simulink model "SignalGen"  (R2014a)
settings: Solver=ode45  StartTime=0.0  StopTime=inf  RelTol=1e-3
undefined symbols (not defined in the file or in its folder): f, Tsample
libraries: dspxfrm3 x3, dspsrcs4 x2, dsparch4 x1, dspsigops x1, commnoisgen2 x1
settings Model: Creator=pHysiX  LastModifiedBy=MrBigBear
settings DebuggingCC: UnderspecifiedInitializationDetection=Classic  StateNameClashWarn=warning

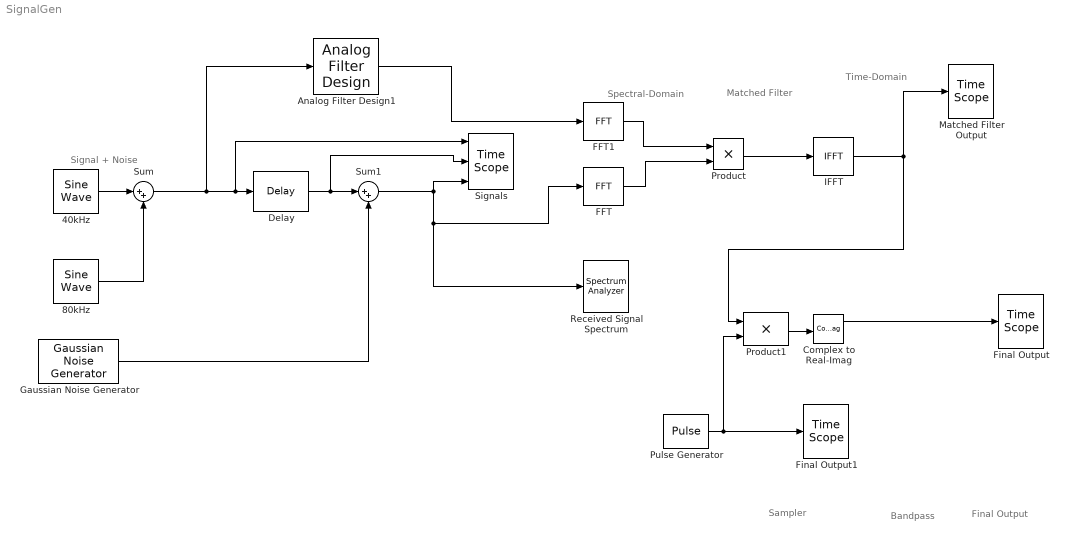
== system SignalGen ==
  note: Signal + Noise
  note: Final Output
  note: Bandpass
  note: Sampler
  note: Time-Domain
  note: Matched Filter
  note: Spectral-Domain
  40kHz : dspsrcs4/Sine Wave  Amplitude=1  Frequency=f  Phase=0  SampleMode=Discrete  OutComplex=Real  CompMethod=Trigonometric fcn  TableSize=Speed  SampleTime=Tsample  SamplesPerFrame=1  ResetState=Restart at time zero  dataType=double  wordLen=16  udDataType=sfix(16)  fracBitsMode=Best precision  numFracBits=15  OutDataTypeStr=double  LastOutDataTypeStr=double
  80kHz : dspsrcs4/Sine Wave  Amplitude=0.5  Frequency=f*2  Phase=0  SampleMode=Discrete  OutComplex=Real  CompMethod=Trigonometric fcn  TableSize=Speed  SampleTime=Tsample/2  SamplesPerFrame=1  ResetState=Restart at time zero  dataType=double  wordLen=16  udDataType=sfix(16)  fracBitsMode=Best precision  numFracBits=15  OutDataTypeStr=double  LastOutDataTypeStr=double
  Analog Filter Design1 : dsparch4/Analog Filter Design  method=Butterworth  filttype=Bandpass  N=8  Wlo=2*pi*39E3  Whi=2*pi*41E3  Rp=2  Rs=40
  Complex to Real-Imag : ComplexToRealImag
  Delay : dspsigops/Delay  dly_unit=Samples  delay=delay  ic_detail=off  dif_ic_for_ch=off  dif_ic_for_dly=off  ic=0  reset_popup=None
  FFT : dspxfrm3/FFT  CompMethod=Table lookup  TableOpt=NEW  TableOptActive=Speed  BitRevOrder=off  InheritFFTLength=on  FFTLength=64  WrapInput=on  RowConvenienceOn=on  FFTImplementation=Auto  SkipNorm=off  firstCoeffDataTypeStr=Inherit: Same word length as input  firstCoeffLastDataTypeStr=Inherit: Same word length as input  outputMin=[]  outputMax=[]  roundingMode=Floor  overflowMode=off
  FFT1 : dspxfrm3/FFT  CompMethod=Table lookup  TableOpt=NEW  TableOptActive=Speed  BitRevOrder=off  InheritFFTLength=on  FFTLength=64  WrapInput=on  RowConvenienceOn=on  FFTImplementation=Auto  SkipNorm=off  firstCoeffDataTypeStr=Inherit: Same word length as input  firstCoeffLastDataTypeStr=Inherit: Same word length as input  outputMin=[]  outputMax=[]  roundingMode=Floor  overflowMode=off
  Final Output : TimeScope  DefaultConfigurationName=spbscopes.TimeScopeBlockCfg
  Final Output1 : TimeScope  DefaultConfigurationName=spbscopes.TimeScopeBlockCfg
  Gaussian Noise Generator : commnoisgen2/Gaussian Noise Generator  m=0  d=1  s=41  Ts=Tsample  frameBased=off  sampPerFrame=1  orient=off  outDataType=double
  IFFT : dspxfrm3/IFFT  CompMethod=Table lookup  TableOpt=NEW  TableOptActive=Speed  BitRevOrder=off  cs_in=off  SkipNorm=on  InheritFFTLength=on  FFTLength=64  WrapInput=on  mode=Complex  outSamplingMode=Sample based  RowConvenienceOn=on  FFTImplementation=Auto  firstCoeffDataTypeStr=Inherit: Same word length as input  firstCoeffLastDataTypeStr=Inherit: Same word length as input  outputMin=[]  outputMax=[]  roundingMode=Nearest  overflowMode=off
  Matched Filter Output : TimeScope  DefaultConfigurationName=spbscopes.TimeScopeBlockCfg
  Product : Product
  Product1 : Product  SaturateOnIntegerOverflow=on  OutDataTypeStr=Inherit: Same as first input
  Pulse Generator : DiscretePulseGenerator  Amplitude=10000  Period=1  SampleTime=Tsample*40
  Received Signal Spectrum : SpectrumAnalyzer
  Signals : TimeScope  NumInputPorts=3  DefaultConfigurationName=spbscopes.TimeScopeBlockCfg
  Sum : Sum  Inputs=|++
  Sum1 : Sum  Inputs=|++
  wires:
  40kHz/1 -> Sum/1
  Delay/1 -> Sum1/1, Signals/2
  Sum/1 -> Analog Filter Design1/1, Delay/1, Signals/1
  80kHz/1 -> Sum/2
  FFT/1 -> Product/2
  FFT1/1 -> Product/1
  Product/1 -> IFFT/1
  IFFT/1 -> Product1/1, Matched Filter Output/1
  Complex to Real-Imag/1 -> Final Output/1
  Pulse Generator/1 -> Final Output1/1, Product1/2
  Product1/1 -> Complex to Real-Imag/1
  Gaussian Noise Generator/1 -> Sum1/2
  Sum1/1 -> Received Signal Spectrum/1, FFT/1, Signals/3
  Analog Filter Design1/1 -> FFT1/1
